simulink model "Kemalettin_KARA_1806A004_HW2"  (R2022a)
settings: Solver=VariableStepAuto  StartTime=0.0  StopTime=10  RelTol=1e-3
libraries: ee_lib x30, fl_lib x12, nesl_utility x4
settings Model: Creator=Cuvan Kanbur  LastModifiedBy=Kemalettin
settings SolverCC: AlgebraicLoopSolver=TrustRegion
settings DebuggingCC: UnconnectedInputMsg=warning  UnconnectedOutputMsg=warning  UnconnectedLineMsg=warning  SFMachineParentedDataDiag=warning
settings RTWCC: DLArmComputeVersion=19.05

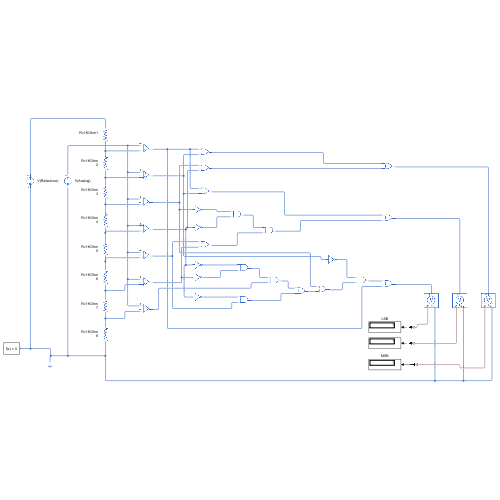
[thumbnail: Simulink's stored preview of the top-level diagram]
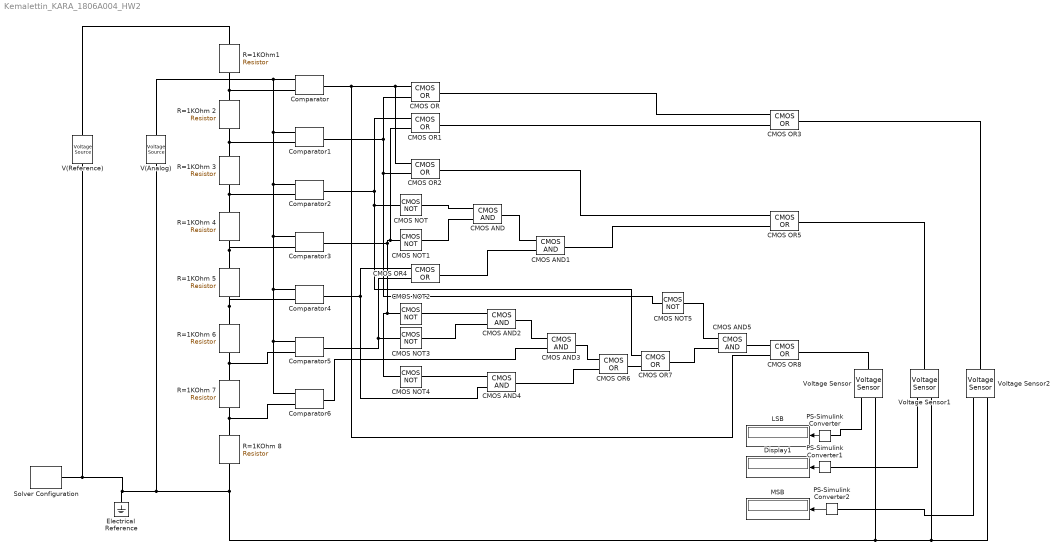
== system Kemalettin_KARA_1806A004_HW2 ==
  CMOS AND{,1..5} (6 alike) : ee_lib/Integrated Circuits/Logic/CMOS AND  V_IL=0.01 V  V_IH=1 V  C_IN=5 pF  output_type=1  V_OL=0 V  V_OH=1 V  V_CC=5 V  V_meas=5 V  R_OUT=25 Ohm  R_OH=[25, 250] Ohm  I_OH=63 mA  R_OL=[30, 800] Ohm  I_OL=-45 mA  Delay=25 ns  Ron=5 Ohm  Vf=0.6 V  output_state=1
      settings: SourceProductBaseCode=PS  InternalSimscapePortConfiguration="{\"Bottom\":[],\"Left\":[{\"id\":\"A\",\"label\":\"\",\"type\":\"foundation.electrical.electrical\"},{\"id\":\"B\",\"label\":\"\",\"type\":\"foundation.electrical.electrical\"}],\"Right\":[{\"id\":\"J\",\"label\":\"\",\"type\":\"foundation.electrical.electrical\"}],\"Top\":[]}"
  CMOS NOT{,1..5} (6 alike) : ee_lib/Integrated Circuits/Logic/CMOS NOT  V_IL=0.01 V  V_IH=1 V  C_IN=5 pF  output_type=1  V_OL=0 V  V_OH=1 V  V_CC=5 V  V_meas=5 V  R_OUT=25 Ohm  R_OH=[25, 250] Ohm  I_OH=63 mA  R_OL=[30, 800] Ohm  I_OL=-45 mA  Delay=25 ns  Ron=5 Ohm  Vf=0.6 V  output_state=1
      settings: SourceProductBaseCode=PS  InternalSimscapePortConfiguration="{\"Bottom\":[],\"Left\":[{\"id\":\"A\",\"label\":\"\",\"type\":\"foundation.electrical.electrical\"}],\"Right\":[{\"id\":\"J\",\"label\":\"\",\"type\":\"foundation.electrical.electrical\"}],\"Top\":[]}"
  CMOS OR{,1..8} (9 alike) : ee_lib/Integrated Circuits/Logic/CMOS OR  V_IL=0.01 V  V_IH=1 V  C_IN=5 pF  output_type=1  V_OL=0 V  V_OH=1 V  V_CC=5 V  V_meas=5 V  R_OUT=25 Ohm  R_OH=[25, 250] Ohm  I_OH=63 mA  R_OL=[30, 800] Ohm  I_OL=-45 mA  Delay=25 ns  Ron=5 Ohm  Vf=0.6 V  output_state=1
      settings: SourceProductBaseCode=PS  InternalSimscapePortConfiguration="{\"Bottom\":[],\"Left\":[{\"id\":\"A\",\"label\":\"\",\"type\":\"foundation.electrical.electrical\"},{\"id\":\"B\",\"label\":\"\",\"type\":\"foundation.electrical.electrical\"}],\"Right\":[{\"id\":\"J\",\"label\":\"\",\"type\":\"foundation.electrical.electrical\"}],\"Top\":[]}"
  Comparator{,1..6} (7 alike) : ee_lib/Integrated Circuits/Comparator  V_OS=5 mV  C_IN=0 pF  V_OL=0 V  V_OH=5 V  R_OUT=50 Ohm  Delay=0 s
      settings: SourceProductBaseCode=PS  InternalSimscapePortConfiguration="{\"Bottom\":[],\"Left\":[{\"id\":\"p\",\"label\":\"+\",\"type\":\"foundation.electrical.electrical\"},{\"id\":\"n\",\"label\":\"-\",\"type\":\"foundation.electrical.electrical\"}],\"Right\":[{\"id\":\"J\",\"label\":\"\",\"type\":\"foundation.electrical.electrical\"}],\"Top\":[]}"
  Display1 : Display
  Electrical Reference : fl_lib/Electrical/Electrical Elements/Electrical Reference
      settings: SourceProductBaseCode=PW,SS,VE
  LSB : Display
  MSB : Display
  PS-Simulink Converter : nesl_utility/PS-Simulink Converter  PhysicalDomain=network_engine_domain  SubClassName=ps_output  LeftPortType=input  RightPortType=output  PseudoPeriodic=off  Frequencies=[]  VectorFormat=1-D array  Unit=inherit  AffineConversion=off
      settings: SourceProductBaseCode=SS,PW,VE
  PS-Simulink Converter1 : nesl_utility/PS-Simulink Converter  PhysicalDomain=network_engine_domain  SubClassName=ps_output  LeftPortType=input  RightPortType=output  PseudoPeriodic=off  Frequencies=[]  VectorFormat=1-D array  Unit=inherit  AffineConversion=off
      settings: SourceProductBaseCode=SS,PW,VE
  PS-Simulink Converter2 : nesl_utility/PS-Simulink Converter  PhysicalDomain=network_engine_domain  SubClassName=ps_output  LeftPortType=input  RightPortType=output  PseudoPeriodic=off  Frequencies=[]  VectorFormat=1-D array  Unit=inherit  AffineConversion=off
      settings: SourceProductBaseCode=SS,PW,VE
  R=1KOhm {2..8} (7 alike) : fl_lib/Electrical/Electrical Elements/Resistor  R=1 kOhm  i_specify=off  i_priority=None  i=0 A  i_nominal_specify=off  i_nominal_unit=A  i_nominal_value=1  v_specify=off  v_priority=None  v=0 V  v_nominal_specify=off  v_nominal_unit=V  v_nominal_value=1
      settings: SourceProductBaseCode=PW,SS,VE
  "R=1KOhm1 " : fl_lib/Electrical/Electrical Elements/Resistor  R=1 kOhm  i_specify=off  i_priority=None  i=0 A  i_nominal_specify=off  i_nominal_unit=A  i_nominal_value=1  v_specify=off  v_priority=None  v=0 V  v_nominal_specify=off  v_nominal_unit=V  v_nominal_value=1
      settings: SourceProductBaseCode=PW,SS,VE
  Solver Configuration : nesl_utility/Solver Configuration  PhysicalDomain=network_engine_domain  SubClassName=solver  LeftPortType=input  RightPortType=generic  Tones=[]  Harmonics=[]  SimulateNoise=off  Profile=off  UseLocalSampling=off  EnableSwitchedLinearOptims=on  FrequencyDomain=off  UseCCode=off  RelTol=0.001  AbsTol=1e-06  MinStep=1e-09  ToWorkspace=off  RevertToSquareIcSolve=off  NumHomotopyIterations=100  PhasorMode=off  PhasorModeNumHarmonics=1  IndexReductionMethod=DerivativeReplacement  DoDC=off  ResidualTolerance=1e-09  UseLocalSolver=off  LocalSolverChoice=NE_BACKWARD_EULER_ADVANCER  LocalSolverSampleTime=0.001  DoFixedCost=off  MaxNonlinIter=3  MaxModeIter=2  ComputeImpulses=off  ImpulseIterations=2  LinearAlgebra=auto  LinearAlgebraNumThread=0  EquationFormulation=NE_TIME_EF  DelaysMemoryBudget=1024  AutomaticFiltering=on  FilteringTimeConstant=0.001  PartitionStorageMethod=AS_NEEDED  PartitionMemoryBudget=1024  PartitionMethod=ROBUST
      settings: SourceProductBaseCode=SS,PW,VE
  V(Analog) : ee_lib/Sources/Voltage Source  dc_voltage=4.55 V  ac_voltage=0 V  ac_shift=0 rad  ac_frequency=60 Hz  noise_mode=0  PSD=0 V^2/Hz  repeatability=1  auto_seed=1734789456  user_seed=0  sample_time=1e-3 s  i_specify=off  i_priority=None  i=0 A  i_nominal_specify=off  i_nominal_unit=A  i_nominal_value=1  v_specify=off  v_priority=None  v=0 V  v_nominal_specify=off  v_nominal_unit=V  v_nominal_value=1
  V(Reference) : ee_lib/Sources/Voltage Source  dc_voltage=5 V  ac_voltage=0 V  ac_shift=0 rad  ac_frequency=60 Hz  noise_mode=0  PSD=0 V^2/Hz  repeatability=1  auto_seed=3497326697  user_seed=0  sample_time=1e-3 s  i_specify=off  i_priority=None  i=0 A  i_nominal_specify=off  i_nominal_unit=A  i_nominal_value=1  v_specify=off  v_priority=None  v=0 V  v_nominal_specify=off  v_nominal_unit=V  v_nominal_value=1
  Voltage Sensor : fl_lib/Electrical/Electrical Sensors/Voltage Sensor
      settings: SourceProductBaseCode=PW,SS,VE
  Voltage Sensor1 : fl_lib/Electrical/Electrical Sensors/Voltage Sensor
      settings: SourceProductBaseCode=PW,SS,VE
  Voltage Sensor2 : fl_lib/Electrical/Electrical Sensors/Voltage Sensor
      settings: SourceProductBaseCode=PW,SS,VE
  wires:
  PS-Simulink Converter/1 -> LSB/1
  PS-Simulink Converter1/1 -> Display1/1
  PS-Simulink Converter2/1 -> MSB/1
  connections:
  R=1KOhm 2/LConn1 -- Comparator/LConn2 -- "R=1KOhm1 "/RConn1
  R=1KOhm 3/LConn1 -- Comparator1/LConn2 -- R=1KOhm 2/RConn1
  R=1KOhm 4/LConn1 -- Comparator2/LConn2 -- R=1KOhm 3/RConn1
  R=1KOhm 5/LConn1 -- Comparator3/LConn2 -- R=1KOhm 4/RConn1
  R=1KOhm 6/LConn1 -- Comparator4/LConn2 -- R=1KOhm 5/RConn1
  R=1KOhm 7/LConn1 -- Comparator5/LConn2 -- R=1KOhm 6/RConn1
  R=1KOhm 8/LConn1 -- Comparator6/LConn2 -- R=1KOhm 7/RConn1
  R=1KOhm 8/RConn1 -- Voltage Sensor/RConn2 -- Voltage Sensor1/RConn2 -- Voltage Sensor2/RConn2 -- V(Analog)/RConn1 -- V(Reference)/RConn1 -- Solver Configuration/RConn1 -- Electrical Reference/LConn1
  V(Reference)/LConn1 -- "R=1KOhm1 "/LConn1
  Comparator/LConn1 -- Comparator1/LConn1 -- Comparator6/LConn1 -- Comparator5/LConn1 -- Comparator4/LConn1 -- Comparator3/LConn1 -- Comparator2/LConn1 -- V(Analog)/LConn1
  Comparator/RConn1 -- CMOS OR/LConn1 -- CMOS OR2/LConn1 -- CMOS OR8/LConn2
  CMOS OR3/LConn1 -- CMOS OR/RConn1
  CMOS OR1/RConn1 -- CMOS OR3/LConn2
  CMOS NOT/RConn1 -- CMOS AND/LConn1
  CMOS NOT1/RConn1 -- CMOS AND/LConn2
  CMOS AND1/LConn1 -- CMOS AND/RConn1
  CMOS OR4/RConn1 -- CMOS AND1/LConn2
  CMOS OR5/LConn2 -- CMOS AND1/RConn1
  CMOS OR5/LConn1 -- CMOS OR2/RConn1
  CMOS OR2/LConn2 -- CMOS OR/LConn2 -- Comparator1/RConn1 -- CMOS NOT5/LConn1
  CMOS NOT2/RConn1 -- CMOS AND2/LConn1
  CMOS NOT3/RConn1 -- CMOS AND2/LConn2
  CMOS AND3/LConn1 -- CMOS AND2/RConn1
  CMOS AND3/LConn2 -- Comparator6/RConn1
  CMOS AND4/LConn1 -- CMOS NOT4/RConn1
  CMOS AND4/LConn2 -- Comparator4/RConn1 -- CMOS OR4/LConn1
  CMOS OR6/LConn1 -- CMOS AND3/RConn1
  CMOS OR6/LConn2 -- CMOS AND4/RConn1
  CMOS OR7/LConn2 -- CMOS OR6/RConn1
  CMOS OR7/LConn1 -- CMOS NOT/LConn1 -- Comparator2/RConn1 -- CMOS OR1/LConn1
  CMOS AND5/LConn1 -- CMOS NOT5/RConn1
  CMOS AND5/LConn2 -- CMOS OR7/RConn1
  CMOS OR8/LConn1 -- CMOS AND5/RConn1
  CMOS NOT4/LConn1 -- CMOS OR1/LConn2 -- CMOS NOT1/LConn1 -- Comparator3/RConn1 -- CMOS NOT2/LConn1
  CMOS OR4/LConn2 -- Comparator5/RConn1 -- CMOS NOT3/LConn1
  Voltage Sensor/LConn1 -- CMOS OR8/RConn1
  Voltage Sensor1/LConn1 -- CMOS OR5/RConn1
  Voltage Sensor2/LConn1 -- CMOS OR3/RConn1
  PS-Simulink Converter/LConn1 -- Voltage Sensor/RConn1
  PS-Simulink Converter1/LConn1 -- Voltage Sensor1/RConn1
  Voltage Sensor2/RConn1 -- PS-Simulink Converter2/LConn1
